simulink model "Regulation_pid"  (Simulink 10.1)
settings: Solver=VariableStepAuto  StartTime=0.0  StopTime=1000  RelTol=1e-3
values from neighbouring files (symbols this model uses):
  b = 3.2 * 10^-10    (= 3.2e-10)    [VariableDrone.m]
  d = 7.9 * 10^-12    (= 7.9e-12)    [VariableDrone.m]
  Fwz = 0    [VariableDrone.m]
  Ix = 1.4 * 10^-5    (= 1.4e-05)    [VariableDrone.m]
  Iy = 1.43 * 10^-5    (= 1.43e-05)    [VariableDrone.m]
  Iz = 2.17 * 10^-5    (= 2.17e-05)    [VariableDrone.m]
  l = 0.04    [VariableDrone.m]
  m = 0.033    [VariableDrone.m]
  Twx = 0    [VariableDrone.m]
  Twy = 0    [VariableDrone.m]
  Twz = 0    [VariableDrone.m]
undefined symbols (not defined in the file or in its folder): Phi, Psi, Theta, w_point
settings Model: Creator=Selim  LastModifiedBy=Selim
settings DataIOCC: SaveFormat=Dataset  ReturnWorkspaceOutputs=on
settings OptimizationCC: LifeSpan=auto
settings DebuggingCC: UnderspecifiedInitializationDetection=Simplified  MergeDetectMultiDrivingBlocksExec=error  SFUnexpectedBacktrackingDiag=error  SFNoUnconditionalDefaultTransitionDiag=error  SFExecutionAtInitializationDiag=warning  ArithmeticOperatorsInVariantConditions=error
settings HardwareCC: ProdBitPerPointer=64  ProdBitPerSizeT=64  ProdBitPerPtrDiffT=64  ProdLargestAtomicFloat=Float  ProdIntDivRoundTo=Zero  ProdEndianess=LittleEndian  ProdWordSize=64  ProdHWDeviceType=Intel->x86-64 (Windows64)
settings ModelReferenceCC: PropagateSignalLabelsOutOfModel=on
settings SFSimCC: SimUseLocalCustomCode=on  CustomCodeUndefinedFunction=FilterOut
settings RTWCC: RTWUseLocalCustomCode=on
settings CodeAppCC: StateflowObjectComments=off
settings GRTTargetCC: TargetLangStandard=C99 (ISO)  CombineOutputUpdateFcns=on  GRTInterface=off
settings ConfigComp: CovMetricSettings=dwe  CovHtmlReporting=off  CovSaveCumulativeToWorkspaceVar=off  CovSaveSingleToWorkspaceVar=off  CovExternalEMLEnable=on

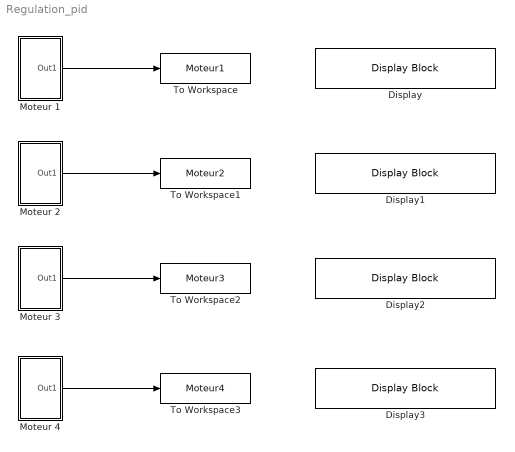
== system Regulation_pid ==
  Display : DisplayBlock  LabelPosition=Hide  Format=short  Transparency=1  GridColor=DataTag1
  Display1 : DisplayBlock  LabelPosition=Hide  Format=short  Transparency=1  GridColor=DataTag3
  Display2 : DisplayBlock  LabelPosition=Hide  Format=short  Transparency=1  GridColor=DataTag5
  Display3 : DisplayBlock  LabelPosition=Hide  Format=short  Transparency=1  GridColor=DataTag7
  Moteur 1 : Subsystem
  Moteur 2 : Subsystem
  Moteur 3 : Subsystem
  Moteur 4 : Subsystem
  To Workspace : ToWorkspace  VariableName=Moteur1  SampleTime=-1
  To Workspace1 : ToWorkspace  VariableName=Moteur2  SampleTime=-1
  To Workspace2 : ToWorkspace  VariableName=Moteur3  SampleTime=-1
  To Workspace3 : ToWorkspace  VariableName=Moteur4  SampleTime=-1
  wires:
  Moteur 1/1(Out1) -> To Workspace/1
  Moteur 4/1(Out1) -> To Workspace3/1
  Moteur 3/1(Out1) -> To Workspace2/1
  Moteur 2/1(Out1) -> To Workspace1/1

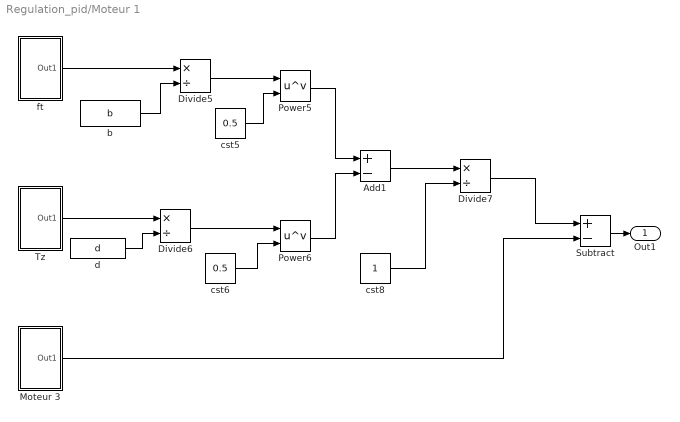
== system Regulation_pid/Moteur 1 ==
  Add1 : Sum  Inputs=+-
  Divide5 : Product  Inputs=*/
  Divide6 : Product  Inputs=*/
  Divide7 : Product  Inputs=*/
  Moteur 3 : Subsystem
  Power5 : Math  Operator=pow  SaturateOnIntegerOverflow=on
  Power6 : Math  Operator=pow  SaturateOnIntegerOverflow=on
  Subtract : Sum  Inputs=+-
  Tz : Subsystem
  b : Constant  Value=b
  cst5 : Constant  Value=0.5
  cst6 : Constant  Value=0.5
  cst8 : Constant
  d : Constant  Value=d
  ft : Subsystem
  Out1 : Outport
  wires:
  Divide6/1 -> Power6/1
  Subtract/1 -> Out1/1
  Add1/1 -> Divide7/1
  Moteur 3/1(Out1) -> Subtract/2
  cst6/1 -> Power6/2
  d/1 -> Divide6/2
  Tz/1(Out1) -> Divide6/1
  ft/1(Out1) -> Divide5/1
  b/1 -> Divide5/2
  Power6/1 -> Add1/2
  Power5/1 -> Add1/1
  cst8/1 -> Divide7/2
  cst5/1 -> Power5/2
  Divide5/1 -> Power5/1
  Divide7/1 -> Subtract/1

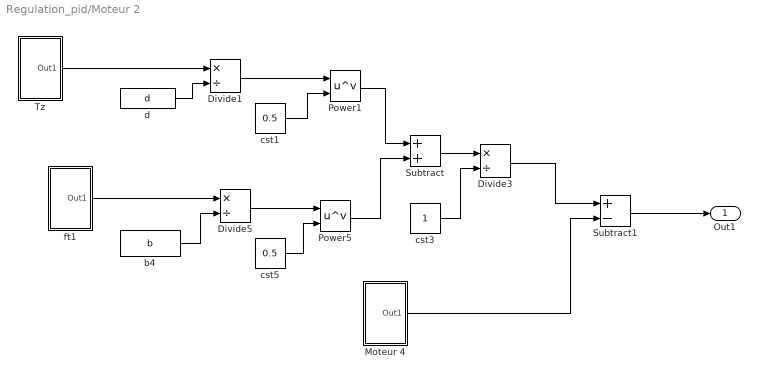
== system Regulation_pid/Moteur 2 ==
  Divide1 : Product  Inputs=*/
  Divide3 : Product  Inputs=*/
  Divide5 : Product  Inputs=*/
  Moteur 4 : Subsystem
  Power1 : Math  Operator=pow  SaturateOnIntegerOverflow=on
  Power5 : Math  Operator=pow  SaturateOnIntegerOverflow=on
  Subtract : Sum
  Subtract1 : Sum  Inputs=+-
  Tz : Subsystem
  b4 : Constant  Value=b
  cst1 : Constant  Value=0.5
  cst3 : Constant
  cst5 : Constant  Value=0.5
  d : Constant  Value=d
  ft1 : Subsystem
  Out1 : Outport
  wires:
  d/1 -> Divide1/2
  Tz/1(Out1) -> Divide1/1
  cst1/1 -> Power1/2
  Divide1/1 -> Power1/1
  Power1/1 -> Subtract/1
  Divide5/1 -> Power5/1
  cst5/1 -> Power5/2
  b4/1 -> Divide5/2
  ft1/1(Out1) -> Divide5/1
  Power5/1 -> Subtract/2
  Subtract/1 -> Divide3/1
  cst3/1 -> Divide3/2
  Subtract1/1 -> Out1/1
  Divide3/1 -> Subtract1/1
  Moteur 4/1(Out1) -> Subtract1/2

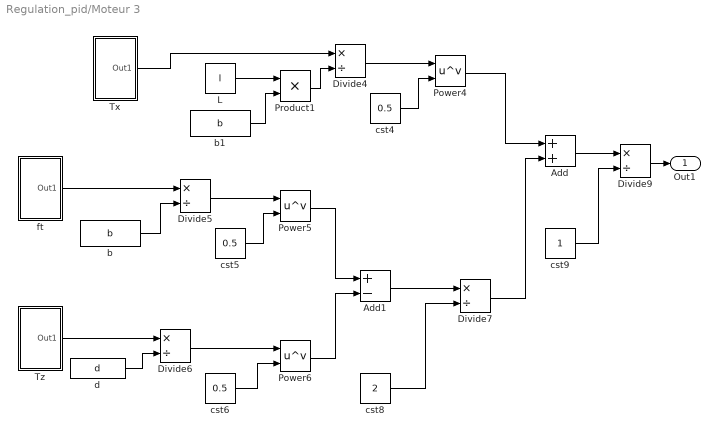
== system Regulation_pid/Moteur 3 ==
  Add : Sum
  Add1 : Sum  Inputs=+-
  Divide{4..7,9} (5 alike) : Product  Inputs=*/
  L : Constant  Value=l
  Power4 : Math  Operator=pow  SaturateOnIntegerOverflow=on
  Power5 : Math  Operator=pow  SaturateOnIntegerOverflow=on
  Power6 : Math  Operator=pow  SaturateOnIntegerOverflow=on
  Product1 : Product
  Tx : Subsystem
  Tz : Subsystem
  b : Constant  Value=b
  b1 : Constant  Value=b
  cst4 : Constant  Value=0.5
  cst5 : Constant  Value=0.5
  cst6 : Constant  Value=0.5
  cst8 : Constant  Value=2
  cst9 : Constant
  d : Constant  Value=d
  ft : Subsystem
  Out1 : Outport
  wires:
  Add1/1 -> Divide7/1
  cst6/1 -> Power6/2
  b1/1 -> Product1/2
  cst8/1 -> Divide7/2
  Add/1 -> Divide9/1
  Divide7/1 -> Add/2
  Power5/1 -> Add1/1
  b/1 -> Divide5/2
  Divide6/1 -> Power6/1
  Power6/1 -> Add1/2
  cst4/1 -> Power4/2
  Product1/1 -> Divide4/2
  Divide4/1 -> Power4/1
  Tz/1(Out1) -> Divide6/1
  d/1 -> Divide6/2
  L/1 -> Product1/1
  Tx/1(Out1) -> Divide4/1
  cst5/1 -> Power5/2
  Divide5/1 -> Power5/1
  Power4/1 -> Add/1
  ft/1(Out1) -> Divide5/1
  cst9/1 -> Divide9/2
  Divide9/1 -> Out1/1

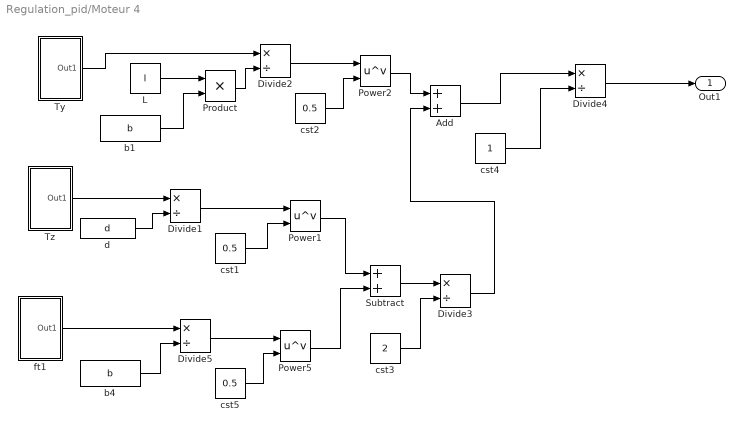
== system Regulation_pid/Moteur 4 ==
  Add : Sum
  Divide{1..5} (5 alike) : Product  Inputs=*/
  L : Constant  Value=l
  Power1 : Math  Operator=pow  SaturateOnIntegerOverflow=on
  Power2 : Math  Operator=pow  SaturateOnIntegerOverflow=on
  Power5 : Math  Operator=pow  SaturateOnIntegerOverflow=on
  Product : Product
  Subtract : Sum
  Ty : Subsystem
  Tz : Subsystem
  b1 : Constant  Value=b
  b4 : Constant  Value=b
  cst1 : Constant  Value=0.5
  cst2 : Constant  Value=0.5
  cst3 : Constant  Value=2
  cst4 : Constant
  cst5 : Constant  Value=0.5
  d : Constant  Value=d
  ft1 : Subsystem
  Out1 : Outport
  wires:
  Power2/1 -> Add/1
  b1/1 -> Product/2
  Product/1 -> Divide2/2
  cst2/1 -> Power2/2
  L/1 -> Product/1
  Divide2/1 -> Power2/1
  Ty/1(Out1) -> Divide2/1
  Subtract/1 -> Divide3/1
  Power5/1 -> Subtract/2
  cst3/1 -> Divide3/2
  d/1 -> Divide1/2
  cst1/1 -> Power1/2
  Tz/1(Out1) -> Divide1/1
  Divide1/1 -> Power1/1
  b4/1 -> Divide5/2
  ft1/1(Out1) -> Divide5/1
  cst5/1 -> Power5/2
  Divide5/1 -> Power5/1
  Power1/1 -> Subtract/1
  Divide3/1 -> Add/2
  Add/1 -> Divide4/1
  cst4/1 -> Divide4/2
  Divide4/1 -> Out1/1

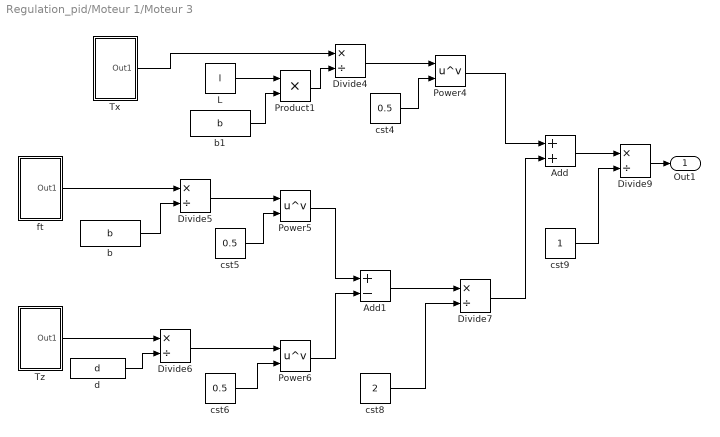
== system Regulation_pid/Moteur 1/Moteur 3 ==
  Add : Sum
  Add1 : Sum  Inputs=+-
  Divide{4..7,9} (5 alike) : Product  Inputs=*/
  L : Constant  Value=l
  Power4 : Math  Operator=pow  SaturateOnIntegerOverflow=on
  Power5 : Math  Operator=pow  SaturateOnIntegerOverflow=on
  Power6 : Math  Operator=pow  SaturateOnIntegerOverflow=on
  Product1 : Product
  Tx : Subsystem
  Tz : Subsystem
  b : Constant  Value=b
  b1 : Constant  Value=b
  cst4 : Constant  Value=0.5
  cst5 : Constant  Value=0.5
  cst6 : Constant  Value=0.5
  cst8 : Constant  Value=2
  cst9 : Constant
  d : Constant  Value=d
  ft : Subsystem
  Out1 : Outport
  wires:
  Add1/1 -> Divide7/1
  cst6/1 -> Power6/2
  b1/1 -> Product1/2
  cst8/1 -> Divide7/2
  Add/1 -> Divide9/1
  Divide7/1 -> Add/2
  Power5/1 -> Add1/1
  b/1 -> Divide5/2
  Divide6/1 -> Power6/1
  Power6/1 -> Add1/2
  cst4/1 -> Power4/2
  Product1/1 -> Divide4/2
  Divide4/1 -> Power4/1
  Tz/1(Out1) -> Divide6/1
  d/1 -> Divide6/2
  L/1 -> Product1/1
  Tx/1(Out1) -> Divide4/1
  cst5/1 -> Power5/2
  Divide5/1 -> Power5/1
  Power4/1 -> Add/1
  ft/1(Out1) -> Divide5/1
  cst9/1 -> Divide9/2
  Divide9/1 -> Out1/1

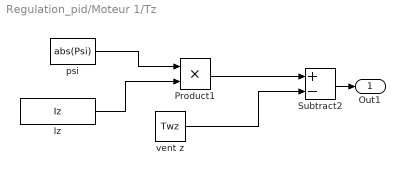
== system Regulation_pid/Moteur 1/Tz ==
  Iz : Constant  Value=Iz
  Product1 : Product
  Subtract2 : Sum  Inputs=+-
  psi : Constant  Value=abs(Psi)
  vent z : Constant  Value=Twz
  Out1 : Outport
  wires:
  Product1/1 -> Subtract2/1
  psi/1 -> Product1/1
  Iz/1 -> Product1/2
  vent z/1 -> Subtract2/2
  Subtract2/1 -> Out1/1

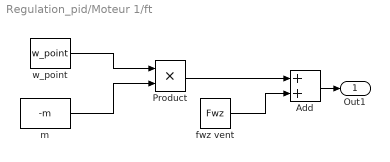
== system Regulation_pid/Moteur 1/ft ==
  Add : Sum
  Product : Product
  fwz vent : Constant  Value=Fwz
  m : Constant  Value=-m
  w_point : Constant  Value=w_point
  Out1 : Outport
  wires:
  m/1 -> Product/2
  Add/1 -> Out1/1
  Product/1 -> Add/1
  fwz vent/1 -> Add/2
  w_point/1 -> Product/1

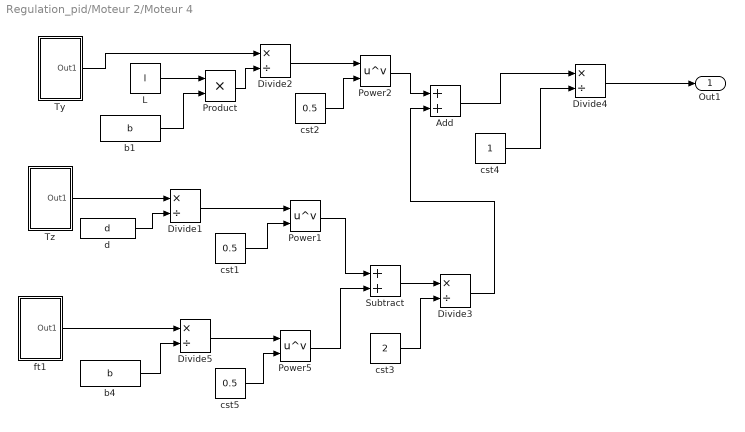
== system Regulation_pid/Moteur 2/Moteur 4 ==
  Add : Sum
  Divide{1..5} (5 alike) : Product  Inputs=*/
  L : Constant  Value=l
  Power1 : Math  Operator=pow  SaturateOnIntegerOverflow=on
  Power2 : Math  Operator=pow  SaturateOnIntegerOverflow=on
  Power5 : Math  Operator=pow  SaturateOnIntegerOverflow=on
  Product : Product
  Subtract : Sum
  Ty : Subsystem
  Tz : Subsystem
  b1 : Constant  Value=b
  b4 : Constant  Value=b
  cst1 : Constant  Value=0.5
  cst2 : Constant  Value=0.5
  cst3 : Constant  Value=2
  cst4 : Constant
  cst5 : Constant  Value=0.5
  d : Constant  Value=d
  ft1 : Subsystem
  Out1 : Outport
  wires:
  Power2/1 -> Add/1
  b1/1 -> Product/2
  Product/1 -> Divide2/2
  cst2/1 -> Power2/2
  L/1 -> Product/1
  Divide2/1 -> Power2/1
  Ty/1(Out1) -> Divide2/1
  Subtract/1 -> Divide3/1
  Power5/1 -> Subtract/2
  cst3/1 -> Divide3/2
  d/1 -> Divide1/2
  cst1/1 -> Power1/2
  Tz/1(Out1) -> Divide1/1
  Divide1/1 -> Power1/1
  b4/1 -> Divide5/2
  ft1/1(Out1) -> Divide5/1
  cst5/1 -> Power5/2
  Divide5/1 -> Power5/1
  Power1/1 -> Subtract/1
  Divide3/1 -> Add/2
  Add/1 -> Divide4/1
  cst4/1 -> Divide4/2
  Divide4/1 -> Out1/1

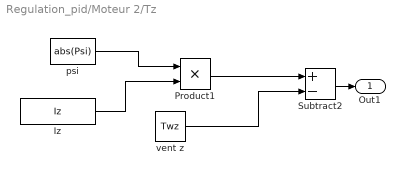
== system Regulation_pid/Moteur 2/Tz ==
  Iz : Constant  Value=Iz
  Product1 : Product
  Subtract2 : Sum  Inputs=+-
  psi : Constant  Value=abs(Psi)
  vent z : Constant  Value=Twz
  Out1 : Outport
  wires:
  Product1/1 -> Subtract2/1
  psi/1 -> Product1/1
  Iz/1 -> Product1/2
  vent z/1 -> Subtract2/2
  Subtract2/1 -> Out1/1

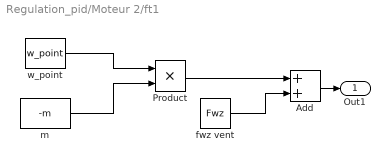
== system Regulation_pid/Moteur 2/ft1 ==
  Add : Sum
  Product : Product
  fwz vent : Constant  Value=Fwz
  m : Constant  Value=-m
  w_point : Constant  Value=w_point
  Out1 : Outport
  wires:
  m/1 -> Product/2
  Add/1 -> Out1/1
  Product/1 -> Add/1
  fwz vent/1 -> Add/2
  w_point/1 -> Product/1

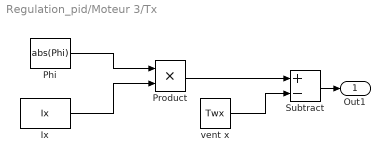
== system Regulation_pid/Moteur 3/Tx ==
  Ix : Constant  Value=Ix
  Phi : Constant  Value=abs(Phi)
  Product : Product
  Subtract : Sum  Inputs=+-
  vent x : Constant  Value=Twx
  Out1 : Outport
  wires:
  Product/1 -> Subtract/1
  Subtract/1 -> Out1/1
  Ix/1 -> Product/2
  vent x/1 -> Subtract/2
  Phi/1 -> Product/1

== system Regulation_pid/Moteur 3/Tz ==
  Iz : Constant  Value=Iz
  Product1 : Product
  Subtract2 : Sum  Inputs=+-
  psi : Constant  Value=abs(Psi)
  vent z : Constant  Value=Twz
  Out1 : Outport
  wires:
  Product1/1 -> Subtract2/1
  psi/1 -> Product1/1
  Iz/1 -> Product1/2
  vent z/1 -> Subtract2/2
  Subtract2/1 -> Out1/1

== system Regulation_pid/Moteur 3/ft ==
  Add : Sum
  Product : Product
  fwz vent : Constant  Value=Fwz
  m : Constant  Value=-m
  w_point : Constant  Value=w_point
  Out1 : Outport
  wires:
  m/1 -> Product/2
  Add/1 -> Out1/1
  Product/1 -> Add/1
  fwz vent/1 -> Add/2
  w_point/1 -> Product/1

== system Regulation_pid/Moteur 4/Ty ==
  Iy : Constant  Value=Iy
  Product2 : Product
  Subtract1 : Sum  Inputs=+-
  theta : Constant  Value=abs(Theta)
  vent y : Constant  Value=Twy
  Out1 : Outport
  wires:
  vent y/1 -> Subtract1/2
  theta/1 -> Product2/1
  Subtract1/1 -> Out1/1
  Iy/1 -> Product2/2
  Product2/1 -> Subtract1/1

== system Regulation_pid/Moteur 4/Tz ==
  Iz : Constant  Value=Iz
  Product1 : Product
  Subtract2 : Sum  Inputs=+-
  psi : Constant  Value=abs(Psi)
  vent z : Constant  Value=Twz
  Out1 : Outport
  wires:
  Product1/1 -> Subtract2/1
  psi/1 -> Product1/1
  Iz/1 -> Product1/2
  vent z/1 -> Subtract2/2
  Subtract2/1 -> Out1/1

== system Regulation_pid/Moteur 4/ft1 ==
  Add : Sum
  Product : Product
  fwz vent : Constant  Value=Fwz
  m : Constant  Value=-m
  w_point : Constant  Value=w_point
  Out1 : Outport
  wires:
  m/1 -> Product/2
  Add/1 -> Out1/1
  Product/1 -> Add/1
  fwz vent/1 -> Add/2
  w_point/1 -> Product/1

== system Regulation_pid/Moteur 1/Moteur 3/Tx ==
  Ix : Constant  Value=Ix
  Phi : Constant  Value=abs(Phi)
  Product : Product
  Subtract : Sum  Inputs=+-
  vent x : Constant  Value=Twx
  Out1 : Outport
  wires:
  Product/1 -> Subtract/1
  Subtract/1 -> Out1/1
  Ix/1 -> Product/2
  vent x/1 -> Subtract/2
  Phi/1 -> Product/1

== system Regulation_pid/Moteur 1/Moteur 3/Tz ==
  Iz : Constant  Value=Iz
  Product1 : Product
  Subtract2 : Sum  Inputs=+-
  psi : Constant  Value=abs(Psi)
  vent z : Constant  Value=Twz
  Out1 : Outport
  wires:
  Product1/1 -> Subtract2/1
  psi/1 -> Product1/1
  Iz/1 -> Product1/2
  vent z/1 -> Subtract2/2
  Subtract2/1 -> Out1/1

== system Regulation_pid/Moteur 1/Moteur 3/ft ==
  Add : Sum
  Product : Product
  fwz vent : Constant  Value=Fwz
  m : Constant  Value=-m
  w_point : Constant  Value=w_point
  Out1 : Outport
  wires:
  m/1 -> Product/2
  Add/1 -> Out1/1
  Product/1 -> Add/1
  fwz vent/1 -> Add/2
  w_point/1 -> Product/1

== system Regulation_pid/Moteur 2/Moteur 4/Ty ==
  Iy : Constant  Value=Iy
  Product2 : Product
  Subtract1 : Sum  Inputs=+-
  theta : Constant  Value=abs(Theta)
  vent y : Constant  Value=Twy
  Out1 : Outport
  wires:
  vent y/1 -> Subtract1/2
  theta/1 -> Product2/1
  Subtract1/1 -> Out1/1
  Iy/1 -> Product2/2
  Product2/1 -> Subtract1/1

== system Regulation_pid/Moteur 2/Moteur 4/Tz ==
  Iz : Constant  Value=Iz
  Product1 : Product
  Subtract2 : Sum  Inputs=+-
  psi : Constant  Value=abs(Psi)
  vent z : Constant  Value=Twz
  Out1 : Outport
  wires:
  Product1/1 -> Subtract2/1
  psi/1 -> Product1/1
  Iz/1 -> Product1/2
  vent z/1 -> Subtract2/2
  Subtract2/1 -> Out1/1

== system Regulation_pid/Moteur 2/Moteur 4/ft1 ==
  Add : Sum
  Product : Product
  fwz vent : Constant  Value=Fwz
  m : Constant  Value=-m
  w_point : Constant  Value=w_point
  Out1 : Outport
  wires:
  m/1 -> Product/2
  Add/1 -> Out1/1
  Product/1 -> Add/1
  fwz vent/1 -> Add/2
  w_point/1 -> Product/1
